simulink model "ohc_nl_boltzman_function"  (R2020b)
settings: Solver=FixedStepDiscrete  StartTime=0.0  StopTime=stopTime  FixedStep=2.0833333333333333e-05  RelTol=1e-3
values from neighbouring files (symbols this model uses):
  s0 = 12.0    (= 12)    [modelparameters.m]    (also in ohc_nl_boltzman_parameters.m)
  s1 = 5.0    (= 5)    [modelparameters.m]    (also in ohc_nl_boltzman_parameters.m)
  shift = 1.0/(1.0+ohcasym)    (= 0.125)    [modelparameters.m]    (also in ohc_nl_boltzman_parameters.m = 1.0/(1.0+ohcasym))
  x0 = s0*log((1.0/shift-1)/(1+exp(x1/s1)))    [modelparameters.m]    (also in ohc_nl_boltzman_parameters.m)
  x1 = 5.0    (= 5)    [modelparameters.m]    (also in ohc_nl_boltzman_parameters.m)
settings Model: Creator=Ross  LastModifiedBy=conno
settings DataIOCC: SaveOutput=off  SaveTime=off  ReturnWorkspaceOutputs=off
settings OptimizationCC: BlockReduction=off  ConditionallyExecuteInputs=off  DefaultParameterBehavior=Inlined
settings DebuggingCC: ReadBeforeWriteMsg=DisableAll  WriteAfterWriteMsg=DisableAll  WriteAfterReadMsg=DisableAll  AlgebraicLoopMsg=error  MultiTaskDSMMsg=none  SingleTaskRateTransMsg=error  PregeneratedLibrarySubsystemCodeDiagnostic=none  ArithmeticOperatorsInVariantConditions=warning
settings HardwareCC: ProdBitPerPointer=32  ProdBitPerSizeT=32  ProdBitPerPtrDiffT=32  ProdLargestAtomicFloat=None  ProdIntDivRoundTo=Undefined  ProdEndianess=Unspecified  ProdWordSize=32  ProdHWDeviceType=ASIC/FPGA->ASIC/FPGA  TargetBitPerPointer=64  TargetBitPerSizeT=64  TargetBitPerPtrDiffT=64  TargetLongLongMode=on  TargetIntDivRoundTo=Zero  TargetEndianess=LittleEndian  TargetWordSize=64  TargetHWDeviceType=Custom Processor->MATLAB Host Computer  ProdEqTarget=off
settings ModelReferenceCC: UpdateModelReferenceTargets=IfOutOfDate
settings SFSimCC: SFSimEcho=off  SimUseLocalCustomCode=off  CustomCodeUndefinedFunction=UseInterfaceOnly
settings RTWCC: RTWUseLocalCustomCode=off

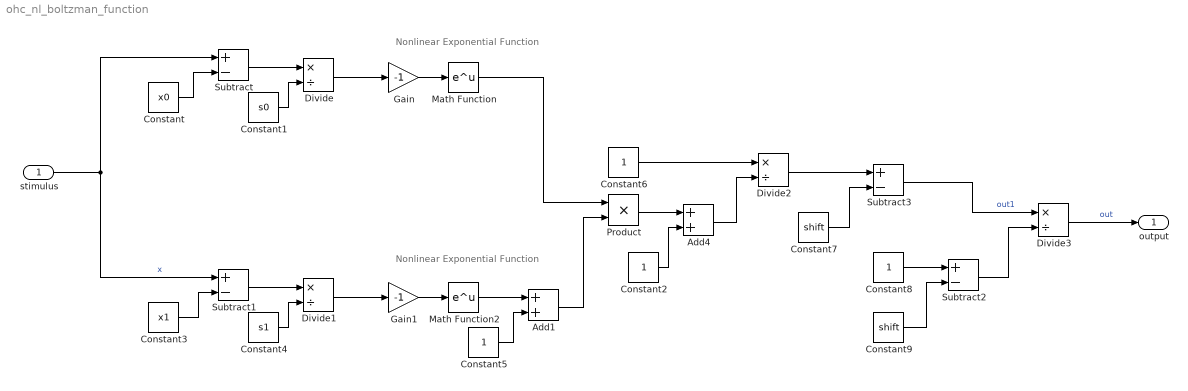
== system ohc_nl_boltzman_function ==
  note: Nonlinear Exponential Function
  note: Nonlinear Exponential Function
  stimulus : Inport  OutDataTypeStr=single  PortDimensions=1  SampleTime=[2.0833333333333333e-05,0]
  Add1 : Sum
  Add4 : Sum
  Constant : Constant  Value=x0  OutDataTypeStr=single  SampleTime=-1
  Constant1 : Constant  Value=s0  OutDataTypeStr=single  SampleTime=-1
  Constant{2,5..6,8} (4 alike) : Constant  OutDataTypeStr=single  SampleTime=-1
  Constant3 : Constant  Value=x1  OutDataTypeStr=single  SampleTime=-1
  Constant4 : Constant  Value=s1  OutDataTypeStr=single  SampleTime=-1
  Constant7 : Constant  Value=shift  OutDataTypeStr=single  SampleTime=-1
  Constant9 : Constant  Value=shift  OutDataTypeStr=single  SampleTime=-1
  Divide{,1..3} (4 alike) : Product  Inputs=*/  RndMeth=Zero  SaturateOnIntegerOverflow=on
  Gain : Gain  Gain=-1
  Gain1 : Gain  Gain=-1
  Math Function : Math  SignedPower=on  SaturateOnIntegerOverflow=on
  Math Function2 : Math  SignedPower=on  SaturateOnIntegerOverflow=on
  Product : Product
  Subtract{,1..3} (4 alike) : Sum  Inputs=+-
  output : Outport  OutDataTypeStr=single  PortDimensions=1  SampleTime=[2.0833333333333333e-05,0]  VectorParamsAs1DForOutWhenUnconnected=off
  wires:
  Add4/1 -> Divide2/2
  Constant2/1 -> Add4/2
  Product/1 -> Add4/1
  Math Function/1 -> Product/1
  Divide3/1 -> output/1  "out"
  Subtract2/1 -> Divide3/2
  Constant9/1 -> Subtract2/2
  Constant8/1 -> Subtract2/1
  Subtract3/1 -> Divide3/1  "out1"
  Constant7/1 -> Subtract3/2
  Divide2/1 -> Subtract3/1
  Constant6/1 -> Divide2/1
  Add1/1 -> Product/2
  Constant5/1 -> Add1/2
  Math Function2/1 -> Add1/1
  Gain1/1 -> Math Function2/1
  Divide1/1 -> Gain1/1
  Constant4/1 -> Divide1/2
  Subtract1/1 -> Divide1/1
  Constant3/1 -> Subtract1/2
  Gain/1 -> Math Function/1
  Divide/1 -> Gain/1
  Constant1/1 -> Divide/2
  Subtract/1 -> Divide/1
  stimulus/1 -> Subtract1/1, Subtract/1  "x"
  Constant/1 -> Subtract/2
